simulink model "Electrical"  (R2019b)
settings: Solver=VariableStepAuto  StartTime=0.0  StopTime=10.0  RelTol=1e-3
values from neighbouring files (symbols this model uses):
  A = 1    [model_1.m]
  R_LED_max = 75/4    (= 18.75)    [FullSystem.m]
libraries: fl_lib x34, nesl_utility x22, ee_lib x20, eePwmGenerator x4, powerlib x3, electricdrivelib x1
settings Model: Creator=thequ  LastModifiedBy=thequ

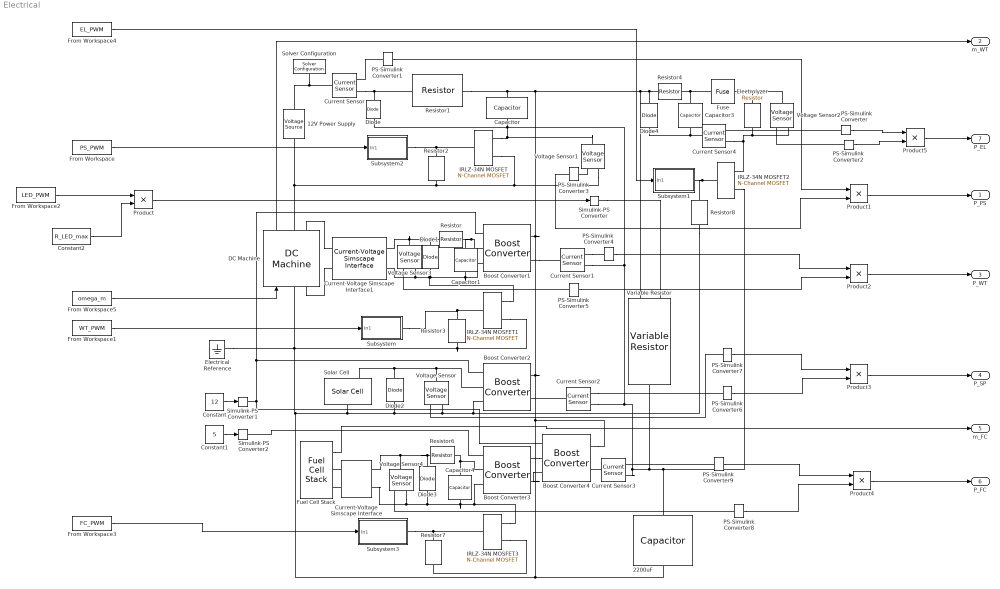
== system Electrical ==
  12V Power Supply : ee_lib/Sources/Voltage Source  dc_voltage=12 V  ac_voltage=0 V  ac_shift=0 rad  ac_frequency=60 Hz  noise_mode=0  PSD=0 V^2/Hz  repeatability=1  auto_seed=3499211588  user_seed=0  sample_time=1e-3 s  i_specify=off  i_priority=None  i=0 A  i_nominal_specify=off  i_nominal_unit=A  i_nominal_value=1  v_specify=off  v_priority=None  v=0 V  v_nominal_specify=off  v_nominal_unit=V  v_nominal_value=1
      settings: SourceProductName=Simscape Electrical
  2200uF : fl_lib/Electrical/Electrical Elements/Capacitor  c=2200 uF  r=1e-6 Ohm  g=0 1/Ohm  i_specify=off  i_priority=None  i=0 A  i_nominal_specify=off  i_nominal_unit=A  i_nominal_value=1  v_specify=off  v_priority=None  v=0 V  v_nominal_specify=off  v_nominal_unit=V  v_nominal_value=1  vc_specify=off  vc_priority=High  vc=0 V  vc_nominal_specify=off  vc_nominal_unit=V  vc_nominal_value=1
  Boost Converter{1..4} (4 alike) : ee_lib/Semiconductors & Converters/Converters/Boost Converter  device_type=2  Vf=0.8 V  Ron=0.001 Ohm  Rds=0.001 Ohm  Goff=1e-5 1/Ohm  Vth=6 V  Vgt=1 V  Vgt_off=-1 V  Ih=1 A  diode_param=0  diode_Vf=0.8 V  diode_Ron=0.001 Ohm  diode_Goff=1e-5 1/Ohm  diode_C=50 nF  diode_iRM=-235 A  diode_iF=300 A  diode_idot=-50 A/us  diode_trr_param=1  diode_trr_factor=3  diode_trr=15 us  diode_Qrr=1500 s*uA  Lf=1e-6 H  Cf=1e-7 F  Rf=1e-6 Ohm  snubber_type=0  Rs=0.1 Ohm  Cs=1e-7 F
      settings: SourceProductName=Simscape Electrical  SourceProductBaseCode=PS  InternalSimscapePortConfiguration="{\"Bottom\":[],\"Left\":[{\"id\":\"G\",\"label\":\"G\",\"type\":\"input\"},{\"id\":\"p1\",\"label\":\"1+\",\"type\":\"foundation.electrical.electrical\"},{\"id\":\"n1\",\"label\":\"1-\",\"type\":\"foundation.electrical.electrical\"}],\"Right\":[{\"id\":\"p2\",\"label\":\"2+\",\"type\":\"foundation.electrical.electrical\"},{\"id\":\"n2\",\"label\":\"2-\",\"type\":\"foundation.electrical.electrical\"}],\"Top\":[]}"
  Capacitor : fl_lib/Electrical/Electrical Elements/Capacitor  c=1000 uF  r=1e-6 Ohm  g=0 1/Ohm  i_specify=off  i_priority=None  i=0 A  i_nominal_specify=off  i_nominal_unit=A  i_nominal_value=1  v_specify=off  v_priority=None  v=0 V  v_nominal_specify=off  v_nominal_unit=V  v_nominal_value=1  vc_specify=off  vc_priority=High  vc=0 V  vc_nominal_specify=off  vc_nominal_unit=V  vc_nominal_value=1
  Capacitor1 : fl_lib/Electrical/Electrical Elements/Capacitor  c=1e-6 F  r=1e-6 Ohm  g=0 1/Ohm  i_specify=off  i_priority=None  i=0 A  i_nominal_specify=off  i_nominal_unit=A  i_nominal_value=1  v_specify=off  v_priority=None  v=0 V  v_nominal_specify=off  v_nominal_unit=V  v_nominal_value=1  vc_specify=off  vc_priority=High  vc=0 V  vc_nominal_specify=off  vc_nominal_unit=V  vc_nominal_value=1
  Capacitor3 : fl_lib/Electrical/Electrical Elements/Capacitor  c=1e-6 F  r=1e-6 Ohm  g=0 1/Ohm  i_specify=off  i_priority=None  i=0 A  i_nominal_specify=off  i_nominal_unit=A  i_nominal_value=1  v_specify=off  v_priority=None  v=0 V  v_nominal_specify=off  v_nominal_unit=V  v_nominal_value=1  vc_specify=off  vc_priority=High  vc=0 V  vc_nominal_specify=off  vc_nominal_unit=V  vc_nominal_value=1
  Capacitor4 : fl_lib/Electrical/Electrical Elements/Capacitor  c=1e-6 F  r=1e-6 Ohm  g=0 1/Ohm  i_specify=off  i_priority=None  i=0 A  i_nominal_specify=off  i_nominal_unit=A  i_nominal_value=1  v_specify=off  v_priority=None  v=0 V  v_nominal_specify=off  v_nominal_unit=V  v_nominal_value=1  vc_specify=off  vc_priority=High  vc=0 V  vc_nominal_specify=off  vc_nominal_unit=V  vc_nominal_value=1
  Constant : Constant  Value=12
  Constant1 : Constant  Value=5
  Constant2 : Constant  Value=R_LED_max
  Current Sensor{,1..4} (5 alike) : fl_lib/Electrical/Electrical Sensors/Current Sensor
  Current-Voltage Simscape Interface : powerlib/Interface Elements/Current-Voltage Simscape Interface  DFT=off  FMode=Low pass filter (continuous)  T=1e-6  Ts=50e-6  i0=0  v0=5  Sd=Specialized Power Systems side  Measurements=off
      settings: SourceProductName=Simscape Electrical  SourceProductBaseCode=PS
  Current-Voltage Simscape Interface1 : powerlib/Interface Elements/Current-Voltage Simscape Interface  DFT=off  FMode=Low pass filter (continuous)  T=1e-6  Ts=50e-6  i0=0  v0=0  Sd=Specialized Power Systems side  Measurements=off
      settings: SourceProductName=Simscape Electrical  SourceProductBaseCode=PS
  DC Machine : powerlib/Machines/DC Machine  PresetModel=No  MechanicalLoad=Speed w  FieldType=Permanent magnet  ShowDetailedParameters=on  MeasurementBus=off  RLa="[0.6  0.012]"  RLf="[ 240  120]"  Laf=1.8  MachineConstant=Torque constant (N.m/A)  Ke=1.8  Kt=0.0283  J=1  Bm=0  Tf=0  w0=1  Ifinit=1  TsPowergui=0  TsBlock=-1
      settings: SourceProductName=Simscape Electrical
  Diode : ee_lib/Semiconductors & Converters/Diode  ModelType=ee.enum.diode.modelType.pwl  Vf=0.6 V  Ron=0.3 Ohm  Goff=1e-8 S  prmExp=ee.enum.diode.expParam.useTwo  I12=[.0137, .545] A  V12=[.6, .7] V  IS=1e-12 A  ec=1  I1=0.0137 A  V1=0.6 V  RS=0 Ohm  Tmeas=25 degC  N_series=1  N_parallel=1  Rz=0.3 Ohm  BV=inf V  C_param=ee.enum.diode.capParam.fixed  CJ=5 pF  CJ0=5 pF  VJ=1 V  Mgrad=0.5  Vvec=[.1, 10, 100] V  Cvec=[3.5, 1, .4] pF  FC=0.5  Q_param=ee.enum.diode.recoveryParam.off  iRM=-7.15 A  iF=4 A  didt=-750 A/us  trr_factor=3  trr=115 ns  Qrr=1500 s*uA  TT=50 ns  tau=100 ns  T_param=ee.enum.diode.temperatureParam.off  IS_T2=1.25e-7 A  I1_T2=0.245 A  V1_T2=0.5 V  Tmeas2=125 degC  EG_param=ee.enum.diode.egapParam.material_si  EG=1.11 eV  XTI_param=ee.enum.diode.xtiParam.pn  XTI=3  dBVdT=0 V/K  Tdevice=25 degC  i_specify=off  i_priority=None  i=0 A  i_nominal_specify=off  i_nominal_unit=A  i_nominal_value=1  v_specify=off  v_priority=None  v=0 V  v_nominal_specify=off  v_nominal_unit=V  v_nominal_value=1  i_capacitor_specify=off  i_capacitor_priority=None  i_capacitor=0 A  i_capacitor_nominal_specify=off  i_capacitor_nominal_unit=A  i_capacitor_nominal_value=1  v_capacitor_specify=off  v_capacitor_priority=None  v_capacitor=0 V  v_capacitor_nominal_specify=off  v_capacitor_nominal_unit=V  v_capacitor_nominal_value=1  power_dissipated_specify=off  power_dissipated_priority=None  power_dissipated=0 W  power_dissipated_nominal_specify=off  power_dissipated_nominal_unit=W  power_dissipated_nominal_value=1  thermal_network_parameterization=ee.enum.thermalNetworkTopology.cauer  Rth=[0, 10] K/W  Rth_Foster=[4, 6] K/W  thermal_mass_parameterization=ee.enum.thermalNetwork.timeconstant  thermal_mass=[0, 1] J/K  thermal_mass_Foster=[1.5, 3] J/K  thermal_time_constant=[0, 10] s  thermal_time_constant_Foster=[6, 18] s  thermal_mass_initial_temperatures=[25, 25] degC
      settings: SourceProductName=Simscape Electrical
  Diode{1..4} (4 alike) : ee_lib/Semiconductors & Converters/Diode  ModelType=ee.enum.diode.modelType.pwl  Vf=0.7 V  Ron=0.3 Ohm  Goff=1e-8 S  prmExp=ee.enum.diode.expParam.useTwo  I12=[.0137, .545] A  V12=[.6, .7] V  IS=1e-12 A  ec=1  I1=0.0137 A  V1=0.6 V  RS=0 Ohm  Tmeas=25 degC  N_series=1  N_parallel=1  Rz=0.3 Ohm  BV=inf V  C_param=ee.enum.diode.capParam.fixed  CJ=5 pF  CJ0=5 pF  VJ=1 V  Mgrad=0.5  Vvec=[.1, 10, 100] V  Cvec=[3.5, 1, .4] pF  FC=0.5  Q_param=ee.enum.diode.recoveryParam.off  iRM=-7.15 A  iF=4 A  didt=-750 A/us  trr_factor=3  trr=115 ns  Qrr=1500 s*uA  TT=50 ns  tau=100 ns  T_param=ee.enum.diode.temperatureParam.off  IS_T2=1.25e-7 A  I1_T2=0.245 A  V1_T2=0.5 V  Tmeas2=125 degC  EG_param=ee.enum.diode.egapParam.material_si  EG=1.11 eV  XTI_param=ee.enum.diode.xtiParam.pn  XTI=3  dBVdT=0 V/K  Tdevice=25 degC  i_specify=off  i_priority=None  i=0 A  i_nominal_specify=off  i_nominal_unit=A  i_nominal_value=1  v_specify=off  v_priority=None  v=0 V  v_nominal_specify=off  v_nominal_unit=V  v_nominal_value=1  i_capacitor_specify=off  i_capacitor_priority=None  i_capacitor=0 A  i_capacitor_nominal_specify=off  i_capacitor_nominal_unit=A  i_capacitor_nominal_value=1  v_capacitor_specify=off  v_capacitor_priority=None  v_capacitor=0 V  v_capacitor_nominal_specify=off  v_capacitor_nominal_unit=V  v_capacitor_nominal_value=1  power_dissipated_specify=off  power_dissipated_priority=None  power_dissipated=0 W  power_dissipated_nominal_specify=off  power_dissipated_nominal_unit=W  power_dissipated_nominal_value=1  thermal_network_parameterization=ee.enum.thermalNetworkTopology.cauer  Rth=[0, 10] K/W  Rth_Foster=[4, 6] K/W  thermal_mass_parameterization=ee.enum.thermalNetwork.timeconstant  thermal_mass=[0, 1] J/K  thermal_mass_Foster=[1.5, 3] J/K  thermal_time_constant=[0, 10] s  thermal_time_constant_Foster=[6, 18] s  thermal_mass_initial_temperatures=[25, 25] degC
      settings: SourceProductName=Simscape Electrical
  Electrical Reference : fl_lib/Electrical/Electrical Elements/Electrical Reference
  Electrolyzer : fl_lib/Electrical/Electrical Elements/Resistor  R=4 Ohm  i_specify=off  i_priority=None  i=0 A  i_nominal_specify=off  i_nominal_unit=A  i_nominal_value=1  v_specify=off  v_priority=None  v=0 V  v_nominal_specify=off  v_nominal_unit=V  v_nominal_value=1
  From Workspace5 : FromWorkspace  VariableName=omega_m  SampleTime=0
  From Workspace : FromWorkspace  VariableName=PS_PWM  SampleTime=0
  From Workspace1 : FromWorkspace  VariableName=WT_PWM  SampleTime=0
  From Workspace2 : FromWorkspace  VariableName=LED_PWM  SampleTime=0
  From Workspace3 : FromWorkspace  VariableName=FC_PWM  SampleTime=0
  From Workspace4 : FromWorkspace  VariableName=EL_PWM  SampleTime=0
  Fuel Cell Stack : electricdrivelib/Extra Sources/Fuel Cell Stack  PresetModel=No (User-Defined)  FcType=0  Detailed=Simplified  Eoc=[2,1]  NomVI=[1,1]  EndVI=[0.9,1.2]  Nc=65  n=55  TOp=65  AirFr=300  SuppPress=[1.5,1]  Comp=[99.95,21,1]  SignX=off  SignY=off  FlowRateH2=off  FlowRateAir=off  SystemTemp=off  SystemPH2=off  SystemPAir=off  FCDyn=off  FC_tau=1  Peak_O2=80  V_Under=10
      settings: SourceProductName=Simscape Electrical  SourceProductBaseCode=PS
  Fuse : ee_lib/Switches & Breakers/Fuse  prm=1  I_rated=1 A  melt_margin=1  T_fuse=0 s  I2t=1 s*A^2  I_vec=[1.9, 2, 2.5, 30] A  t_vec=[10000, 1, .3, .001] s  R_closed=0.01 Ohm  G_open=1e-8 1/Ohm  exposemeasurement=ee.enum.exposemeasurement.hidden
      settings: SourceProductName=Simscape Electrical  SourceProductBaseCode=PS  InternalSimscapePortConfiguration="{\"Bottom\":[],\"Left\":[{\"id\":\"p\",\"label\":\"\",\"type\":\"foundation.electrical.electrical\"}],\"Right\":[{\"id\":\"n\",\"label\":\"\",\"type\":\"foundation.electrical.electrical\"}],\"Top\":[]}"
  IRLZ-34N MOSFET{,1..3} (4 alike) : ee_lib/Semiconductors & Converters/N-Channel MOSFET  parameterization=1  prmDatasheet=1  prmEquCoeff=1  Beta=5.0 A/V^2  Rds=0.046 Ohm  Id=30 A  Vgs=5 V  Vth=1.5 V  lam=0 1/V  Tmeas=25 degC  RS=0.0001 Ohm  RD=0.01 Ohm  C_param=1  C_GS=270 pF  C_GD=80 pF  C_DS=0 pF  C_iss=350 pF  C_rss=80 pF  C_oss=0 pF  C_GS_vec=[270, 300, 290, 280, 295, 255] pF  C_GD_vec=[450, 400, 300, 190, 95, 55] pF  C_DS_vec=[450, 410, 390, 230, 175, 115] pF  C_iss_vec=[720, 700, 590, 470, 390, 310] pF  C_rss_vec=[450, 400, 300, 190, 95, 55] pF  C_oss_vec=[900, 810, 690, 420, 270, 170] pF  C_Vds_vec=[.1, .3, 1, 3, 10, 30] V  V_GS_for_cap_data=0 V  charge_linearity_param=1  C_OX=200 pF  V_C_OX=-0.5 V  IsDiode=0 A  Vbi=0.6 V  n=1  Cj0Diode=0 pF  TT=50e-9 s  dVth_dT=-6 mV/K  Rds_T2=0.037 Ohm  Tmeas2=125 degC  BEXDatasheet=-1.5  BEXEquCoeff=-1.5  etaisDatasheet=3  etaisEquCoeff=3  TdeviceDatasheet=25 degC  TdeviceEquCoeff=25 degC  thermal_network_parameterization=ee.enum.thermalNetworkTopology.cauer  Rth=[0, 10] K/W  Rth_Foster=[4, 6] K/W  thermal_mass_parameterization=ee.enum.thermalNetwork.timeconstant  thermal_mass=[0, 1] J/K  thermal_mass_Foster=[1.5, 3] J/K  thermal_time_constant=[0, 10] s  thermal_time_constant_Foster=[6, 18] s  thermal_mass_initial_temperatures=[25, 25] degC  betaref=18 A/V^2  Vfbref=-1.1 V  gamma=3.5 V^0.50000  phib2ref=1 V  thesatref=0.4 1/V  alpha=0  Vp=5e-2 V  thesrref=0 1/V  m=8  Tref=25 degC  Cox=1500 pF  Cgso=100 pF  Cgdo=14 pF  Rsref=2e-3 Ohm  Rdref=0.17 Ohm  Rgref=8.4 Ohm  Isref=5.2e-13 A  Cj0=480 pF  Tprm=1  etabet=1.3  Stvfb=5e-4 V/K  Stphib=-8.5e-4 V/K  etasat=1.04  etasr=0.65  etar=0.95  etais=3  Tsim=25 degC  T0=[25, 25] degC
      settings: SourceProductName=Simscape Electrical
  PS-Simulink Converter{,1..9} (10 alike) : nesl_utility/PS-Simulink Converter  PhysicalDomain=network_engine_domain  SubClassName=ps_output  LeftPortType=input  RightPortType=output  PseudoPeriodic=off  Frequencies=[]  Unit=inherit  AffineConversion=off
  Product{,1..5} (6 alike) : Product
  Resistor : fl_lib/Electrical/Electrical Elements/Resistor  R=1 Ohm  i_specify=off  i_priority=None  i=0 A  i_nominal_specify=off  i_nominal_unit=A  i_nominal_value=1  v_specify=off  v_priority=None  v=0 V  v_nominal_specify=off  v_nominal_unit=V  v_nominal_value=1
  Resistor1 : fl_lib/Electrical/Electrical Elements/Resistor  R=100 Ohm  i_specify=off  i_priority=None  i=0 A  i_nominal_specify=off  i_nominal_unit=A  i_nominal_value=1  v_specify=off  v_priority=None  v=0 V  v_nominal_specify=off  v_nominal_unit=V  v_nominal_value=1
  Resistor{2..3,7..8} (4 alike) : fl_lib/Electrical/Electrical Elements/Resistor  R=10000 Ohm  i_specify=off  i_priority=None  i=0 A  i_nominal_specify=off  i_nominal_unit=A  i_nominal_value=1  v_specify=off  v_priority=None  v=0 V  v_nominal_specify=off  v_nominal_unit=V  v_nominal_value=1
  Resistor4 : fl_lib/Electrical/Electrical Elements/Resistor  R=1 Ohm  i_specify=off  i_priority=None  i=0 A  i_nominal_specify=off  i_nominal_unit=A  i_nominal_value=1  v_specify=off  v_priority=None  v=0 V  v_nominal_specify=off  v_nominal_unit=V  v_nominal_value=1
  Resistor6 : fl_lib/Electrical/Electrical Elements/Resistor  R=1 Ohm  i_specify=off  i_priority=None  i=0 A  i_nominal_specify=off  i_nominal_unit=A  i_nominal_value=1  v_specify=off  v_priority=None  v=0 V  v_nominal_specify=off  v_nominal_unit=V  v_nominal_value=1
  Simulink-PS Converter : nesl_utility/Simulink-PS Converter  PhysicalDomain=network_engine_domain  SubClassName=ps_input  LeftPortType=input  RightPortType=output  PseudoPeriodic=off  Frequencies=[]  NoiseDistribution=none  NoiseParameters=[]  Unit=1  AffineConversion=off  FilteringAndDerivatives=provide  SimscapeFilterOrder=1  InputFilterTimeConstant=0.001  UdotUserProvided=0
  Simulink-PS Converter1 : nesl_utility/Simulink-PS Converter  PhysicalDomain=network_engine_domain  SubClassName=ps_input  LeftPortType=input  RightPortType=output  PseudoPeriodic=off  Frequencies=[]  NoiseDistribution=none  NoiseParameters=[]  Unit=1  AffineConversion=off  FilteringAndDerivatives=provide  SimscapeFilterOrder=1  InputFilterTimeConstant=0.001  UdotUserProvided=0
  Simulink-PS Converter2 : nesl_utility/Simulink-PS Converter  PhysicalDomain=network_engine_domain  SubClassName=ps_input  LeftPortType=input  RightPortType=output  PseudoPeriodic=off  Frequencies=[]  NoiseDistribution=none  NoiseParameters=[]  Unit=1  AffineConversion=off  FilteringAndDerivatives=provide  SimscapeFilterOrder=1  InputFilterTimeConstant=0.001  UdotUserProvided=0
  Solar Cell : ee_lib/Sources/Solar Cell  prm=1  Isc=7.34 A  Voc=5.5 V  Is=1e-6 A  Is2=0 A  Iph=7.34 A  Ir0=1000 W/m^2  ec=1.5  N2=2  Rs=0 Ohm  Rp=inf Ohm  N_series=1  TIPH1=0 1/K  EG=1.11 eV  TXIS1=3  TXIS2=3  TRS1=0  TRP1=0  Tmeas=25 degC  TFIXED=25 degC  thermal_mass=100 J/K  initial_temperature=25 degC
      settings: SourceProductName=Simscape Electrical  SourceProductBaseCode=PS
  Solver Configuration : nesl_utility/Solver Configuration  PhysicalDomain=network_engine_domain  SubClassName=solver  LeftPortType=input  RightPortType=generic  Tones=[]  Harmonics=[]  SimulateNoise=off  Profile=off  UseLocalSampling=off  EnableSwitchedLinearOptims=on  FrequencyDomain=off  UseCCode=off  RelTol=0.001  AbsTol=1e-06  MinStep=1e-09  ToWorkspace=off  RevertToSquareIcSolve=off  NumHomotopyIterations=100  PhasorMode=off  PhasorModeNumHarmonics=1  DoDC=off  ResidualTolerance=1e-09  UseLocalSolver=off  LocalSolverChoice=NE_BACKWARD_EULER_ADVANCER  LocalSolverSampleTime=0.001  DoFixedCost=off  MaxNonlinIter=3  MaxModeIter=2  LinearAlgebra=auto  EquationFormulation=NE_TIME_EF  DelaysMemoryBudget=1024  AutomaticFiltering=on  FilteringTimeConstant=0.001  PartitionStorageMethod=AS_NEEDED  PartitionMemoryBudget=1024  PartitionMethod=ROBUST
  Subsystem : Subsystem
  Subsystem1 : Subsystem
  Subsystem2 : Subsystem
  Subsystem3 : Subsystem
  Variable Resistor : fl_lib/Electrical/Electrical Elements/Variable Resistor  Rmin=10 Ohm  i_specify=off  i_priority=None  i=0 A  i_nominal_specify=off  i_nominal_unit=A  i_nominal_value=1  v_specify=off  v_priority=None  v=0 V  v_nominal_specify=off  v_nominal_unit=V  v_nominal_value=1
  Voltage Sensor{,1..4} (5 alike) : fl_lib/Electrical/Electrical Sensors/Voltage Sensor
  P_PS : Outport
  m_WT : Outport  Port=2
  P_WT : Outport  Port=3
  P_SP : Outport  Port=4
  m_FC : Outport  Port=5
  P_FC : Outport  Port=6
  P_EL : Outport  Port=7
  wires:
  PS-Simulink Converter1/1 -> Product1/1
  PS-Simulink Converter3/1 -> Product1/2
  Constant/1 -> Simulink-PS Converter1/1
  PS-Simulink Converter5/1 -> Product2/2
  From Workspace1/1 -> Subsystem/1(In1)
  From Workspace/1 -> Subsystem2/1(In1)
  From Workspace3/1 -> Subsystem3/1(In1)
  Fuel Cell Stack/1 -> m_FC/1
  Constant1/1 -> Simulink-PS Converter2/1
  Product/1 -> Simulink-PS Converter/1
  From Workspace4/1 -> Subsystem1/1(In1)
  From Workspace5/1 -> DC Machine/1
  DC Machine/1 -> m_WT/1
  From Workspace2/1 -> Product/1
  Constant2/1 -> Product/2
  Product1/1 -> P_PS/1
  Product2/1 -> P_WT/1
  PS-Simulink Converter4/1 -> Product2/1
  Product3/1 -> P_SP/1
  PS-Simulink Converter6/1 -> Product3/2
  PS-Simulink Converter7/1 -> Product3/1
  PS-Simulink Converter8/1 -> Product4/2
  PS-Simulink Converter9/1 -> Product4/1
  Product4/1 -> P_FC/1
  Product5/1 -> P_EL/1
  PS-Simulink Converter2/1 -> Product5/2
  PS-Simulink Converter/1 -> Product5/1
  connections:
  Resistor1/LConn1 -- Current Sensor/RConn2 -- Diode/RConn1
  Capacitor/RConn1 -- Current Sensor3/RConn2 -- IRLZ-34N MOSFET2/RConn2 -- 2200uF/LConn1 -- Variable Resistor/RConn1 -- Current Sensor2/RConn2 -- Current Sensor1/RConn2 -- IRLZ-34N MOSFET/RConn1 -- Voltage Sensor1/LConn1 -- Diode/LConn1
  Current Sensor/LConn1 -- 12V Power Supply/LConn1 -- Solver Configuration/RConn1
  PS-Simulink Converter1/LConn1 -- Current Sensor/RConn1
  IRLZ-34N MOSFET/LConn1 -- Subsystem2/RConn1 -- Resistor2/LConn1
  PS-Simulink Converter3/LConn1 -- Voltage Sensor1/RConn1
  Resistor/LConn1 -- Voltage Sensor3/LConn1 -- Current-Voltage Simscape Interface1/RConn1 -- Diode1/RConn1
  IRLZ-34N MOSFET1/RConn1 -- Diode1/LConn1 -- Capacitor1/RConn1 -- Boost Converter1/LConn3 -- Voltage Sensor3/RConn2 -- Current-Voltage Simscape Interface1/RConn2
  Resistor/RConn1 -- Capacitor1/LConn1 -- Boost Converter1/LConn2
  Simulink-PS Converter1/RConn1 -- Boost Converter4/LConn1 -- Boost Converter2/LConn1 -- Boost Converter1/LConn1
  PS-Simulink Converter5/LConn1 -- Voltage Sensor3/RConn1
  Resistor1/RConn1 -- Diode4/RConn1 -- Resistor4/LConn1 -- Variable Resistor/LConn2 -- 2200uF/RConn1 -- Voltage Sensor/RConn2 -- Resistor8/RConn1 -- Boost Converter2/LConn3 -- Diode2/LConn1 -- Solar Cell/RConn1 -- IRLZ-34N MOSFET1/RConn2 -- Resistor3/RConn1 -- Electrical Reference/LConn1 -- 12V Power Supply/RConn1 -- Resistor2/RConn1 -- Voltage Sensor1/RConn2 -- IRLZ-34N MOSFET/RConn2 -- Boost Converter4/RConn1 -- Boost Converter2/RConn1 -- Boost Converter1/RConn1 -- Capacitor/LConn1
  Solar Cell/LConn2 -- Voltage Sensor/LConn1 -- Boost Converter2/LConn2 -- Diode2/RConn1
  IRLZ-34N MOSFET1/LConn1 -- Subsystem/RConn1 -- Resistor3/LConn1
  Capacitor4/RConn1 -- IRLZ-34N MOSFET3/RConn1 -- Boost Converter3/LConn3 -- Current-Voltage Simscape Interface/RConn2 -- Voltage Sensor4/RConn2 -- Diode3/LConn1
  IRLZ-34N MOSFET3/RConn2 -- Resistor7/RConn1
  Boost Converter3/LConn2 -- Resistor6/RConn1 -- Capacitor4/LConn1
  Resistor6/LConn1 -- Current-Voltage Simscape Interface/RConn1 -- Voltage Sensor4/LConn1 -- Diode3/RConn1
  Subsystem3/RConn1 -- IRLZ-34N MOSFET3/LConn1 -- Resistor7/LConn1
  Boost Converter3/LConn1 -- Simulink-PS Converter2/RConn1
  Boost Converter3/RConn1 -- Boost Converter4/LConn2
  Boost Converter3/RConn2 -- Boost Converter4/LConn3
  Fuel Cell Stack/RConn1 -- Current-Voltage Simscape Interface/LConn1
  Fuel Cell Stack/RConn2 -- Current-Voltage Simscape Interface/LConn2
  Simulink-PS Converter/RConn1 -- Variable Resistor/LConn1
  Electrolyzer/RConn1 -- IRLZ-34N MOSFET2/RConn1 -- Current Sensor4/RConn2 -- Voltage Sensor2/RConn2
  Capacitor3/LConn1 -- Fuse/LConn1 -- Resistor4/RConn1
  IRLZ-34N MOSFET2/LConn1 -- Resistor8/LConn1 -- Subsystem1/RConn1
  DC Machine/RConn1 -- Current-Voltage Simscape Interface1/LConn1
  DC Machine/LConn1 -- Current-Voltage Simscape Interface1/LConn2
  Boost Converter1/RConn2 -- Current Sensor1/LConn1
  Current Sensor1/RConn1 -- PS-Simulink Converter4/LConn1
  PS-Simulink Converter7/LConn1 -- Voltage Sensor/RConn1
  Current Sensor2/LConn1 -- Boost Converter2/RConn2
  Current Sensor2/RConn1 -- PS-Simulink Converter6/LConn1
  PS-Simulink Converter8/LConn1 -- Voltage Sensor4/RConn1
  Current Sensor3/LConn1 -- Boost Converter4/RConn2
  PS-Simulink Converter9/LConn1 -- Current Sensor3/RConn1
  Fuse/RConn1 -- Voltage Sensor2/LConn1 -- Electrolyzer/LConn1
  Diode4/LConn1 -- Current Sensor4/LConn1 -- Capacitor3/RConn1
  PS-Simulink Converter/LConn1 -- Current Sensor4/RConn1
  PS-Simulink Converter2/LConn1 -- Voltage Sensor2/RConn1

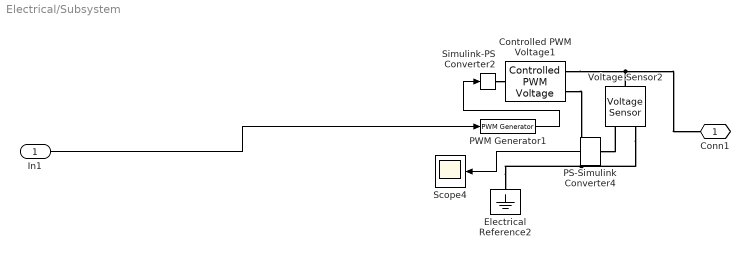
== system Electrical/Subsystem ==
  In1 : Inport
  Controlled PWM Voltage1 : ee_lib/Integrated Circuits/Controlled PWM Voltage  F=490 Hz  TD=0 s  pulse_width_offset=0 s  pulse_min=0 s  Vmin=0 V  Vmax=5 V  Vm=5 V  pwm_or_av=1  event_type=1  sample_time=1e-6 s  u_min=0  u_max=1
      settings: SourceProductName=Simscape Electrical  InternalSimscapePortConfiguration="{\"Bottom\":[],\"Left\":[{\"id\":\"u\",\"label\":\"u\",\"type\":\"input\"}],\"Right\":[{\"id\":\"p2\",\"label\":\"PWM\",\"type\":\"foundation.electrical.electrical\"},{\"id\":\"n2\",\"label\":\"REF\",\"type\":\"foundation.electrical.electrical\"}],\"Top\":[]}"
  Electrical Reference2 : fl_lib/Electrical/Electrical Elements/Electrical Reference
  PS-Simulink Converter4 : nesl_utility/PS-Simulink Converter  PhysicalDomain=network_engine_domain  SubClassName=ps_output  LeftPortType=input  RightPortType=output  PseudoPeriodic=off  Frequencies=[]  Unit=inherit  AffineConversion=off
  PWM Generator1 : eePwmGenerator/PWM Generator  CarrCount=Up  Tper=0.001  Ts=5e-5
      settings: SourceProductName=Simscape Electrical
  Scope4 : Scope
  Simulink-PS Converter2 : nesl_utility/Simulink-PS Converter  PhysicalDomain=network_engine_domain  SubClassName=ps_input  LeftPortType=input  RightPortType=output  PseudoPeriodic=off  Frequencies=[]  NoiseDistribution=none  NoiseParameters=[]  Unit=1  AffineConversion=off  FilteringAndDerivatives=provide  SimscapeFilterOrder=1  InputFilterTimeConstant=0.001  UdotUserProvided=0
  Voltage Sensor2 : fl_lib/Electrical/Electrical Sensors/Voltage Sensor
  Conn1 : PMIOPort  Side=Right
  wires:
  In1/1 -> PWM Generator1/1
  PWM Generator1/1 -> Simulink-PS Converter2/1
  PS-Simulink Converter4/1 -> Scope4/1
  connections:
  PS-Simulink Converter4/LConn1 -- Voltage Sensor2/RConn1
  Electrical Reference2/LConn1 -- Controlled PWM Voltage1/RConn2 -- Voltage Sensor2/RConn2
  Controlled PWM Voltage1/RConn1 -- Conn1/RConn1 -- Voltage Sensor2/LConn1
  Simulink-PS Converter2/RConn1 -- Controlled PWM Voltage1/LConn1

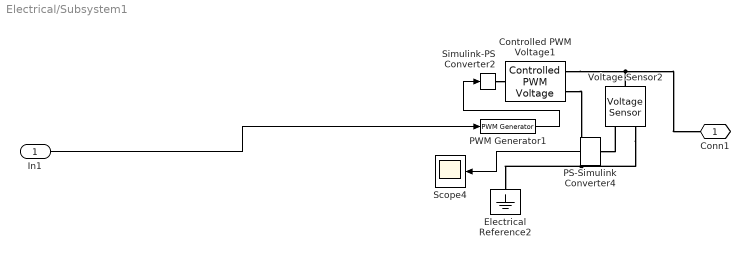
== system Electrical/Subsystem1 ==
  In1 : Inport
  Controlled PWM Voltage1 : ee_lib/Integrated Circuits/Controlled PWM Voltage  F=490 Hz  TD=0 s  pulse_width_offset=0 s  pulse_min=0 s  Vmin=0 V  Vmax=5 V  Vm=5 V  pwm_or_av=1  event_type=1  sample_time=1e-6 s  u_min=0  u_max=1
      settings: SourceProductName=Simscape Electrical  InternalSimscapePortConfiguration="{\"Bottom\":[],\"Left\":[{\"id\":\"u\",\"label\":\"u\",\"type\":\"input\"}],\"Right\":[{\"id\":\"p2\",\"label\":\"PWM\",\"type\":\"foundation.electrical.electrical\"},{\"id\":\"n2\",\"label\":\"REF\",\"type\":\"foundation.electrical.electrical\"}],\"Top\":[]}"
  Electrical Reference2 : fl_lib/Electrical/Electrical Elements/Electrical Reference
  PS-Simulink Converter4 : nesl_utility/PS-Simulink Converter  PhysicalDomain=network_engine_domain  SubClassName=ps_output  LeftPortType=input  RightPortType=output  PseudoPeriodic=off  Frequencies=[]  Unit=inherit  AffineConversion=off
  PWM Generator1 : eePwmGenerator/PWM Generator  CarrCount=Up  Tper=0.001  Ts=5e-5
      settings: SourceProductName=Simscape Electrical
  Scope4 : Scope
  Simulink-PS Converter2 : nesl_utility/Simulink-PS Converter  PhysicalDomain=network_engine_domain  SubClassName=ps_input  LeftPortType=input  RightPortType=output  PseudoPeriodic=off  Frequencies=[]  NoiseDistribution=none  NoiseParameters=[]  Unit=1  AffineConversion=off  FilteringAndDerivatives=provide  SimscapeFilterOrder=1  InputFilterTimeConstant=0.001  UdotUserProvided=0
  Voltage Sensor2 : fl_lib/Electrical/Electrical Sensors/Voltage Sensor
  Conn1 : PMIOPort  Side=Right
  wires:
  In1/1 -> PWM Generator1/1
  PWM Generator1/1 -> Simulink-PS Converter2/1
  PS-Simulink Converter4/1 -> Scope4/1
  connections:
  PS-Simulink Converter4/LConn1 -- Voltage Sensor2/RConn1
  Voltage Sensor2/RConn2 -- Electrical Reference2/LConn1 -- Controlled PWM Voltage1/RConn2
  Voltage Sensor2/LConn1 -- Controlled PWM Voltage1/RConn1 -- Conn1/RConn1
  Simulink-PS Converter2/RConn1 -- Controlled PWM Voltage1/LConn1

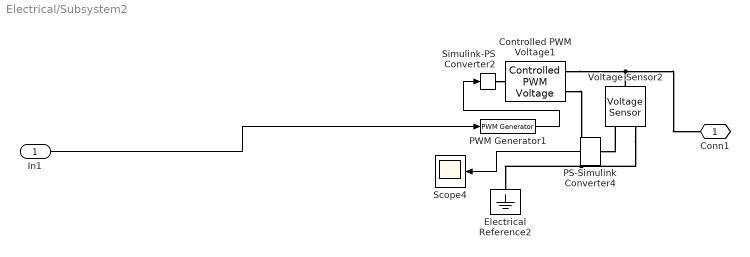
== system Electrical/Subsystem2 ==
  In1 : Inport
  Controlled PWM Voltage1 : ee_lib/Integrated Circuits/Controlled PWM Voltage  F=490 Hz  TD=0 s  pulse_width_offset=0 s  pulse_min=0 s  Vmin=0 V  Vmax=5 V  Vm=5 V  pwm_or_av=1  event_type=1  sample_time=1e-6 s  u_min=0  u_max=1
      settings: SourceProductName=Simscape Electrical  InternalSimscapePortConfiguration="{\"Bottom\":[],\"Left\":[{\"id\":\"u\",\"label\":\"u\",\"type\":\"input\"}],\"Right\":[{\"id\":\"p2\",\"label\":\"PWM\",\"type\":\"foundation.electrical.electrical\"},{\"id\":\"n2\",\"label\":\"REF\",\"type\":\"foundation.electrical.electrical\"}],\"Top\":[]}"
  Electrical Reference2 : fl_lib/Electrical/Electrical Elements/Electrical Reference
  PS-Simulink Converter4 : nesl_utility/PS-Simulink Converter  PhysicalDomain=network_engine_domain  SubClassName=ps_output  LeftPortType=input  RightPortType=output  PseudoPeriodic=off  Frequencies=[]  Unit=inherit  AffineConversion=off
  PWM Generator1 : eePwmGenerator/PWM Generator  CarrCount=Up  Tper=0.001  Ts=5e-5
      settings: SourceProductName=Simscape Electrical
  Scope4 : Scope
  Simulink-PS Converter2 : nesl_utility/Simulink-PS Converter  PhysicalDomain=network_engine_domain  SubClassName=ps_input  LeftPortType=input  RightPortType=output  PseudoPeriodic=off  Frequencies=[]  NoiseDistribution=none  NoiseParameters=[]  Unit=1  AffineConversion=off  FilteringAndDerivatives=provide  SimscapeFilterOrder=1  InputFilterTimeConstant=0.001  UdotUserProvided=0
  Voltage Sensor2 : fl_lib/Electrical/Electrical Sensors/Voltage Sensor
  Conn1 : PMIOPort  Side=Right
  wires:
  In1/1 -> PWM Generator1/1
  PWM Generator1/1 -> Simulink-PS Converter2/1
  PS-Simulink Converter4/1 -> Scope4/1
  connections:
  PS-Simulink Converter4/LConn1 -- Voltage Sensor2/RConn1
  Voltage Sensor2/RConn2 -- Electrical Reference2/LConn1 -- Controlled PWM Voltage1/RConn2
  Voltage Sensor2/LConn1 -- Controlled PWM Voltage1/RConn1 -- Conn1/RConn1
  Simulink-PS Converter2/RConn1 -- Controlled PWM Voltage1/LConn1

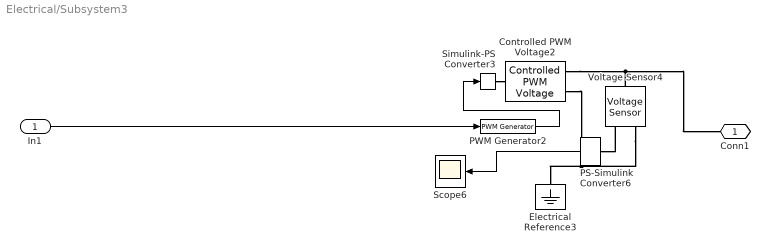
== system Electrical/Subsystem3 ==
  In1 : Inport
  Controlled PWM Voltage2 : ee_lib/Integrated Circuits/Controlled PWM Voltage  F=490 Hz  TD=0 s  pulse_width_offset=0 s  pulse_min=0 s  Vmin=0 V  Vmax=5 V  Vm=5 V  pwm_or_av=1  event_type=1  sample_time=1e-6 s  u_min=0  u_max=1
      settings: SourceProductName=Simscape Electrical  InternalSimscapePortConfiguration="{\"Bottom\":[],\"Left\":[{\"id\":\"u\",\"label\":\"u\",\"type\":\"input\"}],\"Right\":[{\"id\":\"p2\",\"label\":\"PWM\",\"type\":\"foundation.electrical.electrical\"},{\"id\":\"n2\",\"label\":\"REF\",\"type\":\"foundation.electrical.electrical\"}],\"Top\":[]}"
  Electrical Reference3 : fl_lib/Electrical/Electrical Elements/Electrical Reference
  PS-Simulink Converter6 : nesl_utility/PS-Simulink Converter  PhysicalDomain=network_engine_domain  SubClassName=ps_output  LeftPortType=input  RightPortType=output  PseudoPeriodic=off  Frequencies=[]  Unit=inherit  AffineConversion=off
  PWM Generator2 : eePwmGenerator/PWM Generator  CarrCount=Up  Tper=0.001  Ts=5e-5
      settings: SourceProductName=Simscape Electrical
  Scope6 : Scope
  Simulink-PS Converter3 : nesl_utility/Simulink-PS Converter  PhysicalDomain=network_engine_domain  SubClassName=ps_input  LeftPortType=input  RightPortType=output  PseudoPeriodic=off  Frequencies=[]  NoiseDistribution=none  NoiseParameters=[]  Unit=1  AffineConversion=off  FilteringAndDerivatives=provide  SimscapeFilterOrder=1  InputFilterTimeConstant=0.001  UdotUserProvided=0
  Voltage Sensor4 : fl_lib/Electrical/Electrical Sensors/Voltage Sensor
  Conn1 : PMIOPort  Side=Right
  wires:
  PWM Generator2/1 -> Simulink-PS Converter3/1
  In1/1 -> PWM Generator2/1
  PS-Simulink Converter6/1 -> Scope6/1
  connections:
  Voltage Sensor4/LConn1 -- Controlled PWM Voltage2/RConn1 -- Conn1/RConn1
  Voltage Sensor4/RConn2 -- Electrical Reference3/LConn1 -- Controlled PWM Voltage2/RConn2
  PS-Simulink Converter6/LConn1 -- Voltage Sensor4/RConn1
  Simulink-PS Converter3/RConn1 -- Controlled PWM Voltage2/LConn1
